simulink model "LINEARNI_MODEL1"  (R2018b)
settings: Solver=ode45  StartTime=0.0  StopTime=t_sim  RelTol=1e-5
undefined symbols (not defined in the file): du, k, t_step, uh0
settings Model: Creator=student  LastModifiedBy=student

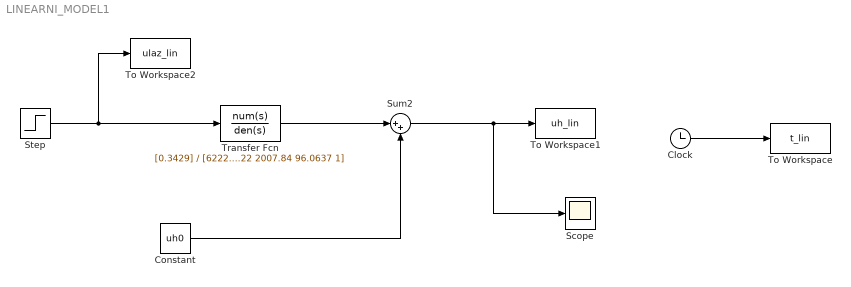
== system LINEARNI_MODEL1 ==
  Clock : Clock
  Constant : Constant  Value=uh0
  Scope : Scope
  Step : Step  Time=t_step  After=k*du  SampleTime=0
  Sum2 : Sum  Inputs=|++
  To Workspace : ToWorkspace  VariableName=t_lin  SampleTime=-1
      settings: Save2DSignal=2-D array (concatenate along first dimension)
  To Workspace1 : ToWorkspace  VariableName=uh_lin  SampleTime=-1
      settings: Save2DSignal=2-D array (concatenate along first dimension)
  To Workspace2 : ToWorkspace  VariableName=ulaz_lin  SampleTime=-1
      settings: Save2DSignal=2-D array (concatenate along first dimension)
  Transfer Fcn : TransferFcn  Numerator=[0.3429]  Denominator=[6222.22 2007.84 96.0637 1]
  wires:
  Step/1 -> To Workspace2/1, Transfer Fcn/1
  Clock/1 -> To Workspace/1
  Transfer Fcn/1 -> Sum2/1
  Constant/1 -> Sum2/2
  Sum2/1 -> To Workspace1/1, Scope/1
